simulink model "kundur_vsg"  (R2025b)
settings: Solver=ode23t  StartTime=0.0  StopTime=10.0  MaxStep=0.001  RelTol=1e-4
libraries: fl_lib x55, ee_lib x53, nesl_utility x17
(part 1 of 2)
settings Model: Creator=27443  LastModifiedBy=27443

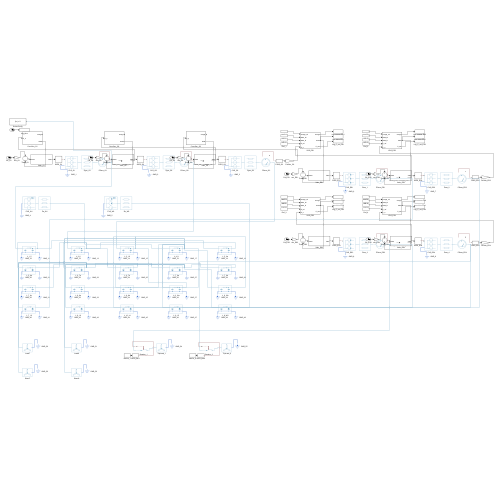
[thumbnail: Simulink's stored preview of the top-level diagram]
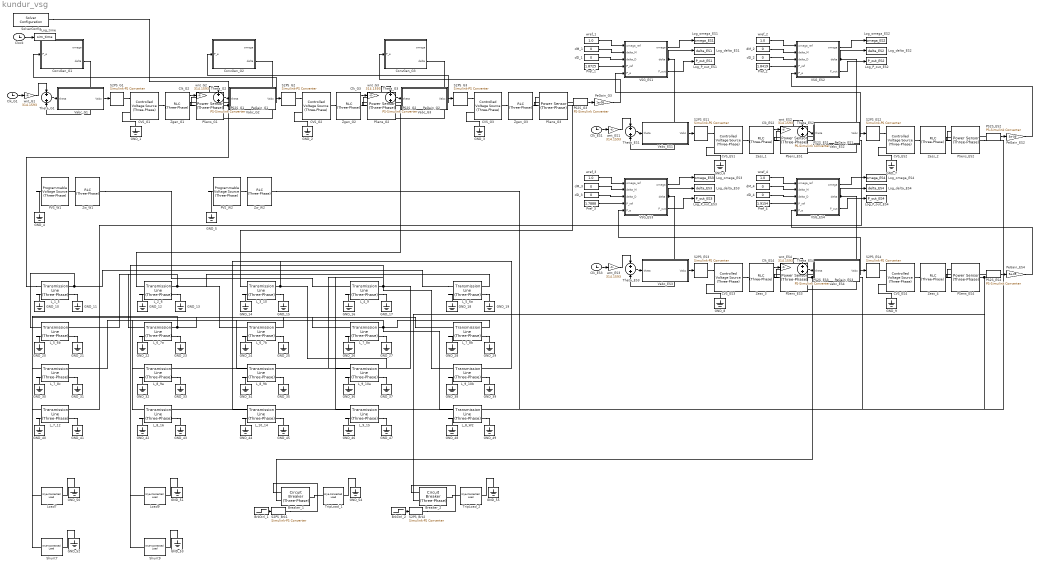
== system kundur_vsg ==
  Breaker_1 : ee_lib/Switches & Breakers/Circuit Breaker (Three-Phase)  R_closed=0.001 Ohm  G_open=1e-6 1/Ohm  threshold=0.5 V  breaker_behavior=ee.enum.switches.breakerBehavior.zeroCrossingEnable
      settings: InternalSimscapePortConfiguration="{\"Bottom\":[],\"Left\":[{\"id\":\"vT\",\"label\":\"vT\",\"type\":\"input\"},{\"id\":\"N1\",\"label\":\"~1\",\"type\":\"foundation.electrical.three_phase\"}],\"Right\":[{\"id\":\"N2\",\"label\":\"~2\",\"type\":\"foundation.electrical.three_phase\"}],\"Top\":[]}"
  Breaker_2 : ee_lib/Switches & Breakers/Circuit Breaker (Three-Phase)  R_closed=0.001 Ohm  G_open=1e-6 1/Ohm  threshold=0.5 V  breaker_behavior=ee.enum.switches.breakerBehavior.zeroCrossingEnable
      settings: InternalSimscapePortConfiguration="{\"Bottom\":[],\"Left\":[{\"id\":\"vT\",\"label\":\"vT\",\"type\":\"input\"},{\"id\":\"N1\",\"label\":\"~1\",\"type\":\"foundation.electrical.three_phase\"}],\"Right\":[{\"id\":\"N2\",\"label\":\"~2\",\"type\":\"foundation.electrical.three_phase\"}],\"Top\":[]}"
  BrkCtrl_1 : Step  Time=100  Before=1  After=0
  BrkCtrl_2 : Step  Time=100
  CVS_ES{1..4} (4 alike) : ee_lib/Sources/Controlled Voltage Source (Three-Phase)  input_option=ee.enum.inputType.instantaneous  FRated=60 Hz
      settings: InternalSimscapePortConfiguration="{\"Bottom\":[],\"Left\":[{\"id\":\"S\",\"label\":\"S\",\"type\":\"input\"},{\"id\":\"n\",\"label\":\"n\",\"type\":\"foundation.electrical.electrical\"}],\"Right\":[{\"id\":\"N\",\"label\":\"~\",\"type\":\"foundation.electrical.three_phase\"}],\"Top\":[]}"
  CVS_G1 : ee_lib/Sources/Controlled Voltage Source (Three-Phase)  input_option=ee.enum.inputType.instantaneous  FRated=60 Hz
      settings: InternalSimscapePortConfiguration="{\"Bottom\":[],\"Left\":[{\"id\":\"S\",\"label\":\"S\",\"type\":\"input\"},{\"id\":\"n\",\"label\":\"n\",\"type\":\"foundation.electrical.electrical\"}],\"Right\":[{\"id\":\"N\",\"label\":\"~\",\"type\":\"foundation.electrical.three_phase\"}],\"Top\":[]}"
  CVS_G2 : ee_lib/Sources/Controlled Voltage Source (Three-Phase)  input_option=ee.enum.inputType.instantaneous  FRated=60 Hz
      settings: InternalSimscapePortConfiguration="{\"Bottom\":[],\"Left\":[{\"id\":\"S\",\"label\":\"S\",\"type\":\"input\"},{\"id\":\"n\",\"label\":\"n\",\"type\":\"foundation.electrical.electrical\"}],\"Right\":[{\"id\":\"N\",\"label\":\"~\",\"type\":\"foundation.electrical.three_phase\"}],\"Top\":[]}"
  CVS_G3 : ee_lib/Sources/Controlled Voltage Source (Three-Phase)  input_option=ee.enum.inputType.instantaneous  FRated=60 Hz
      settings: InternalSimscapePortConfiguration="{\"Bottom\":[],\"Left\":[{\"id\":\"S\",\"label\":\"S\",\"type\":\"input\"},{\"id\":\"n\",\"label\":\"n\",\"type\":\"foundation.electrical.electrical\"}],\"Right\":[{\"id\":\"N\",\"label\":\"~\",\"type\":\"foundation.electrical.three_phase\"}],\"Top\":[]}"
  Clk_ES{1..4} (4 alike) : Clock
  Clk_G1 : Clock
  Clk_G2 : Clock
  Clk_G3 : Clock
  Clock : Clock
  ConvGen_G1 : Subsystem
  ConvGen_G2 : Subsystem
  ConvGen_G3 : Subsystem
  GND_{1..55} (55 alike) : fl_lib/Electrical/Electrical Elements/Electrical Reference
  L_10_14 : ee_lib/Passive/Lines/Transmission Line (Three-Phase)  length=1 km  freq=50 Hz  R=0.01 Ohm/km  L=0.5 mH/km  M=0.1 mH/km  Cl=9 uF/km  Cg=0.1 uF/km  Rm=0 Ohm/km  ModelTwoSections=ee.enum.enable.no  N=1  InterfacePosition=0.5 km  N1sec=1  N2sec=1  Access_ground=ee.enum.enable.no  R_parasitic=1e-6 Ohm  G_parasitic=1e-6 1/Ohm
      settings: InternalSimscapePortConfiguration="{\"Bottom\":[],\"Left\":[{\"id\":\"N1\",\"label\":\"~1\",\"type\":\"foundation.electrical.three_phase\"},{\"id\":\"g1\",\"label\":\"g1\",\"type\":\"foundation.electrical.electrical\"}],\"Right\":[{\"id\":\"N2\",\"label\":\"~2\",\"type\":\"foundation.electrical.three_phase\"},{\"id\":\"g2\",\"label\":\"g2\",\"type\":\"foundation.electrical.electrical\"}],\"Top\":[]}"
  L_1_5 : ee_lib/Passive/Lines/Transmission Line (Three-Phase)  length=5 km  freq=50 Hz  R=0.053 Ohm/km  L=1.41 mH/km  M=0.1 mH/km  Cl=9 uF/km  Cg=0.1 uF/km  Rm=0 Ohm/km  ModelTwoSections=ee.enum.enable.no  N=1  InterfacePosition=0.5 km  N1sec=1  N2sec=1  Access_ground=ee.enum.enable.no  R_parasitic=1e-6 Ohm  G_parasitic=1e-6 1/Ohm
      settings: InternalSimscapePortConfiguration="{\"Bottom\":[],\"Left\":[{\"id\":\"N1\",\"label\":\"~1\",\"type\":\"foundation.electrical.three_phase\"},{\"id\":\"g1\",\"label\":\"g1\",\"type\":\"foundation.electrical.electrical\"}],\"Right\":[{\"id\":\"N2\",\"label\":\"~2\",\"type\":\"foundation.electrical.three_phase\"},{\"id\":\"g2\",\"label\":\"g2\",\"type\":\"foundation.electrical.electrical\"}],\"Top\":[]}"
  L_2_6 : ee_lib/Passive/Lines/Transmission Line (Three-Phase)  length=5 km  freq=50 Hz  R=0.053 Ohm/km  L=1.41 mH/km  M=0.1 mH/km  Cl=9 uF/km  Cg=0.1 uF/km  Rm=0 Ohm/km  ModelTwoSections=ee.enum.enable.no  N=1  InterfacePosition=0.5 km  N1sec=1  N2sec=1  Access_ground=ee.enum.enable.no  R_parasitic=1e-6 Ohm  G_parasitic=1e-6 1/Ohm
      settings: InternalSimscapePortConfiguration="{\"Bottom\":[],\"Left\":[{\"id\":\"N1\",\"label\":\"~1\",\"type\":\"foundation.electrical.three_phase\"},{\"id\":\"g1\",\"label\":\"g1\",\"type\":\"foundation.electrical.electrical\"}],\"Right\":[{\"id\":\"N2\",\"label\":\"~2\",\"type\":\"foundation.electrical.three_phase\"},{\"id\":\"g2\",\"label\":\"g2\",\"type\":\"foundation.electrical.electrical\"}],\"Top\":[]}"
  L_3_10 : ee_lib/Passive/Lines/Transmission Line (Three-Phase)  length=5 km  freq=50 Hz  R=0.053 Ohm/km  L=1.41 mH/km  M=0.1 mH/km  Cl=9 uF/km  Cg=0.1 uF/km  Rm=0 Ohm/km  ModelTwoSections=ee.enum.enable.no  N=1  InterfacePosition=0.5 km  N1sec=1  N2sec=1  Access_ground=ee.enum.enable.no  R_parasitic=1e-6 Ohm  G_parasitic=1e-6 1/Ohm
      settings: InternalSimscapePortConfiguration="{\"Bottom\":[],\"Left\":[{\"id\":\"N1\",\"label\":\"~1\",\"type\":\"foundation.electrical.three_phase\"},{\"id\":\"g1\",\"label\":\"g1\",\"type\":\"foundation.electrical.electrical\"}],\"Right\":[{\"id\":\"N2\",\"label\":\"~2\",\"type\":\"foundation.electrical.three_phase\"},{\"id\":\"g2\",\"label\":\"g2\",\"type\":\"foundation.electrical.electrical\"}],\"Top\":[]}"
  L_4_9 : ee_lib/Passive/Lines/Transmission Line (Three-Phase)  length=5 km  freq=50 Hz  R=0.053 Ohm/km  L=1.41 mH/km  M=0.1 mH/km  Cl=9 uF/km  Cg=0.1 uF/km  Rm=0 Ohm/km  ModelTwoSections=ee.enum.enable.no  N=1  InterfacePosition=0.5 km  N1sec=1  N2sec=1  Access_ground=ee.enum.enable.no  R_parasitic=1e-6 Ohm  G_parasitic=1e-6 1/Ohm
      settings: InternalSimscapePortConfiguration="{\"Bottom\":[],\"Left\":[{\"id\":\"N1\",\"label\":\"~1\",\"type\":\"foundation.electrical.three_phase\"},{\"id\":\"g1\",\"label\":\"g1\",\"type\":\"foundation.electrical.electrical\"}],\"Right\":[{\"id\":\"N2\",\"label\":\"~2\",\"type\":\"foundation.electrical.three_phase\"},{\"id\":\"g2\",\"label\":\"g2\",\"type\":\"foundation.electrical.electrical\"}],\"Top\":[]}"
  L_5_6a : ee_lib/Passive/Lines/Transmission Line (Three-Phase)  length=25 km  freq=50 Hz  R=0.053 Ohm/km  L=1.41 mH/km  M=0.1 mH/km  Cl=9 uF/km  Cg=0.1 uF/km  Rm=0 Ohm/km  ModelTwoSections=ee.enum.enable.no  N=1  InterfacePosition=0.5 km  N1sec=1  N2sec=1  Access_ground=ee.enum.enable.no  R_parasitic=1e-6 Ohm  G_parasitic=1e-6 1/Ohm
      settings: InternalSimscapePortConfiguration="{\"Bottom\":[],\"Left\":[{\"id\":\"N1\",\"label\":\"~1\",\"type\":\"foundation.electrical.three_phase\"},{\"id\":\"g1\",\"label\":\"g1\",\"type\":\"foundation.electrical.electrical\"}],\"Right\":[{\"id\":\"N2\",\"label\":\"~2\",\"type\":\"foundation.electrical.three_phase\"},{\"id\":\"g2\",\"label\":\"g2\",\"type\":\"foundation.electrical.electrical\"}],\"Top\":[]}"
  L_5_6b : ee_lib/Passive/Lines/Transmission Line (Three-Phase)  length=25 km  freq=50 Hz  R=0.053 Ohm/km  L=1.41 mH/km  M=0.1 mH/km  Cl=9 uF/km  Cg=0.1 uF/km  Rm=0 Ohm/km  ModelTwoSections=ee.enum.enable.no  N=1  InterfacePosition=0.5 km  N1sec=1  N2sec=1  Access_ground=ee.enum.enable.no  R_parasitic=1e-6 Ohm  G_parasitic=1e-6 1/Ohm
      settings: InternalSimscapePortConfiguration="{\"Bottom\":[],\"Left\":[{\"id\":\"N1\",\"label\":\"~1\",\"type\":\"foundation.electrical.three_phase\"},{\"id\":\"g1\",\"label\":\"g1\",\"type\":\"foundation.electrical.electrical\"}],\"Right\":[{\"id\":\"N2\",\"label\":\"~2\",\"type\":\"foundation.electrical.three_phase\"},{\"id\":\"g2\",\"label\":\"g2\",\"type\":\"foundation.electrical.electrical\"}],\"Top\":[]}"
  L_6_7a : ee_lib/Passive/Lines/Transmission Line (Three-Phase)  length=10 km  freq=50 Hz  R=0.053 Ohm/km  L=1.41 mH/km  M=0.1 mH/km  Cl=9 uF/km  Cg=0.1 uF/km  Rm=0 Ohm/km  ModelTwoSections=ee.enum.enable.no  N=1  InterfacePosition=0.5 km  N1sec=1  N2sec=1  Access_ground=ee.enum.enable.no  R_parasitic=1e-6 Ohm  G_parasitic=1e-6 1/Ohm
      settings: InternalSimscapePortConfiguration="{\"Bottom\":[],\"Left\":[{\"id\":\"N1\",\"label\":\"~1\",\"type\":\"foundation.electrical.three_phase\"},{\"id\":\"g1\",\"label\":\"g1\",\"type\":\"foundation.electrical.electrical\"}],\"Right\":[{\"id\":\"N2\",\"label\":\"~2\",\"type\":\"foundation.electrical.three_phase\"},{\"id\":\"g2\",\"label\":\"g2\",\"type\":\"foundation.electrical.electrical\"}],\"Top\":[]}"
  L_6_7b : ee_lib/Passive/Lines/Transmission Line (Three-Phase)  length=10 km  freq=50 Hz  R=0.053 Ohm/km  L=1.41 mH/km  M=0.1 mH/km  Cl=9 uF/km  Cg=0.1 uF/km  Rm=0 Ohm/km  ModelTwoSections=ee.enum.enable.no  N=1  InterfacePosition=0.5 km  N1sec=1  N2sec=1  Access_ground=ee.enum.enable.no  R_parasitic=1e-6 Ohm  G_parasitic=1e-6 1/Ohm
      settings: InternalSimscapePortConfiguration="{\"Bottom\":[],\"Left\":[{\"id\":\"N1\",\"label\":\"~1\",\"type\":\"foundation.electrical.three_phase\"},{\"id\":\"g1\",\"label\":\"g1\",\"type\":\"foundation.electrical.electrical\"}],\"Right\":[{\"id\":\"N2\",\"label\":\"~2\",\"type\":\"foundation.electrical.three_phase\"},{\"id\":\"g2\",\"label\":\"g2\",\"type\":\"foundation.electrical.electrical\"}],\"Top\":[]}"
  L_7_12 : ee_lib/Passive/Lines/Transmission Line (Three-Phase)  length=1 km  freq=50 Hz  R=0.01 Ohm/km  L=0.5 mH/km  M=0.1 mH/km  Cl=9 uF/km  Cg=0.1 uF/km  Rm=0 Ohm/km  ModelTwoSections=ee.enum.enable.no  N=1  InterfacePosition=0.5 km  N1sec=1  N2sec=1  Access_ground=ee.enum.enable.no  R_parasitic=1e-6 Ohm  G_parasitic=1e-6 1/Ohm
      settings: InternalSimscapePortConfiguration="{\"Bottom\":[],\"Left\":[{\"id\":\"N1\",\"label\":\"~1\",\"type\":\"foundation.electrical.three_phase\"},{\"id\":\"g1\",\"label\":\"g1\",\"type\":\"foundation.electrical.electrical\"}],\"Right\":[{\"id\":\"N2\",\"label\":\"~2\",\"type\":\"foundation.electrical.three_phase\"},{\"id\":\"g2\",\"label\":\"g2\",\"type\":\"foundation.electrical.electrical\"}],\"Top\":[]}"
  L_7_8a : ee_lib/Passive/Lines/Transmission Line (Three-Phase)  length=110 km  freq=50 Hz  R=0.053 Ohm/km  L=1.41 mH/km  M=0.1 mH/km  Cl=9 uF/km  Cg=0.1 uF/km  Rm=0 Ohm/km  ModelTwoSections=ee.enum.enable.no  N=1  InterfacePosition=0.5 km  N1sec=1  N2sec=1  Access_ground=ee.enum.enable.no  R_parasitic=1e-6 Ohm  G_parasitic=1e-6 1/Ohm
      settings: InternalSimscapePortConfiguration="{\"Bottom\":[],\"Left\":[{\"id\":\"N1\",\"label\":\"~1\",\"type\":\"foundation.electrical.three_phase\"},{\"id\":\"g1\",\"label\":\"g1\",\"type\":\"foundation.electrical.electrical\"}],\"Right\":[{\"id\":\"N2\",\"label\":\"~2\",\"type\":\"foundation.electrical.three_phase\"},{\"id\":\"g2\",\"label\":\"g2\",\"type\":\"foundation.electrical.electrical\"}],\"Top\":[]}"
  L_7_8b : ee_lib/Passive/Lines/Transmission Line (Three-Phase)  length=110 km  freq=50 Hz  R=0.053 Ohm/km  L=1.41 mH/km  M=0.1 mH/km  Cl=9 uF/km  Cg=0.1 uF/km  Rm=0 Ohm/km  ModelTwoSections=ee.enum.enable.no  N=1  InterfacePosition=0.5 km  N1sec=1  N2sec=1  Access_ground=ee.enum.enable.no  R_parasitic=1e-6 Ohm  G_parasitic=1e-6 1/Ohm
      settings: InternalSimscapePortConfiguration="{\"Bottom\":[],\"Left\":[{\"id\":\"N1\",\"label\":\"~1\",\"type\":\"foundation.electrical.three_phase\"},{\"id\":\"g1\",\"label\":\"g1\",\"type\":\"foundation.electrical.electrical\"}],\"Right\":[{\"id\":\"N2\",\"label\":\"~2\",\"type\":\"foundation.electrical.three_phase\"},{\"id\":\"g2\",\"label\":\"g2\",\"type\":\"foundation.electrical.electrical\"}],\"Top\":[]}"
  L_7_8c : ee_lib/Passive/Lines/Transmission Line (Three-Phase)  length=110 km  freq=50 Hz  R=0.053 Ohm/km  L=1.41 mH/km  M=0.1 mH/km  Cl=9 uF/km  Cg=0.1 uF/km  Rm=0 Ohm/km  ModelTwoSections=ee.enum.enable.no  N=1  InterfacePosition=0.5 km  N1sec=1  N2sec=1  Access_ground=ee.enum.enable.no  R_parasitic=1e-6 Ohm  G_parasitic=1e-6 1/Ohm
      settings: InternalSimscapePortConfiguration="{\"Bottom\":[],\"Left\":[{\"id\":\"N1\",\"label\":\"~1\",\"type\":\"foundation.electrical.three_phase\"},{\"id\":\"g1\",\"label\":\"g1\",\"type\":\"foundation.electrical.electrical\"}],\"Right\":[{\"id\":\"N2\",\"label\":\"~2\",\"type\":\"foundation.electrical.three_phase\"},{\"id\":\"g2\",\"label\":\"g2\",\"type\":\"foundation.electrical.electrical\"}],\"Top\":[]}"
  L_8_16 : ee_lib/Passive/Lines/Transmission Line (Three-Phase)  length=1 km  freq=50 Hz  R=0.01 Ohm/km  L=0.5 mH/km  M=0.1 mH/km  Cl=9 uF/km  Cg=0.1 uF/km  Rm=0 Ohm/km  ModelTwoSections=ee.enum.enable.no  N=1  InterfacePosition=0.5 km  N1sec=1  N2sec=1  Access_ground=ee.enum.enable.no  R_parasitic=1e-6 Ohm  G_parasitic=1e-6 1/Ohm
      settings: InternalSimscapePortConfiguration="{\"Bottom\":[],\"Left\":[{\"id\":\"N1\",\"label\":\"~1\",\"type\":\"foundation.electrical.three_phase\"},{\"id\":\"g1\",\"label\":\"g1\",\"type\":\"foundation.electrical.electrical\"}],\"Right\":[{\"id\":\"N2\",\"label\":\"~2\",\"type\":\"foundation.electrical.three_phase\"},{\"id\":\"g2\",\"label\":\"g2\",\"type\":\"foundation.electrical.electrical\"}],\"Top\":[]}"
  L_8_9a : ee_lib/Passive/Lines/Transmission Line (Three-Phase)  length=10 km  freq=50 Hz  R=0.053 Ohm/km  L=1.41 mH/km  M=0.1 mH/km  Cl=9 uF/km  Cg=0.1 uF/km  Rm=0 Ohm/km  ModelTwoSections=ee.enum.enable.no  N=1  InterfacePosition=0.5 km  N1sec=1  N2sec=1  Access_ground=ee.enum.enable.no  R_parasitic=1e-6 Ohm  G_parasitic=1e-6 1/Ohm
      settings: InternalSimscapePortConfiguration="{\"Bottom\":[],\"Left\":[{\"id\":\"N1\",\"label\":\"~1\",\"type\":\"foundation.electrical.three_phase\"},{\"id\":\"g1\",\"label\":\"g1\",\"type\":\"foundation.electrical.electrical\"}],\"Right\":[{\"id\":\"N2\",\"label\":\"~2\",\"type\":\"foundation.electrical.three_phase\"},{\"id\":\"g2\",\"label\":\"g2\",\"type\":\"foundation.electrical.electrical\"}],\"Top\":[]}"
  L_8_9b : ee_lib/Passive/Lines/Transmission Line (Three-Phase)  length=10 km  freq=50 Hz  R=0.053 Ohm/km  L=1.41 mH/km  M=0.1 mH/km  Cl=9 uF/km  Cg=0.1 uF/km  Rm=0 Ohm/km  ModelTwoSections=ee.enum.enable.no  N=1  InterfacePosition=0.5 km  N1sec=1  N2sec=1  Access_ground=ee.enum.enable.no  R_parasitic=1e-6 Ohm  G_parasitic=1e-6 1/Ohm
      settings: InternalSimscapePortConfiguration="{\"Bottom\":[],\"Left\":[{\"id\":\"N1\",\"label\":\"~1\",\"type\":\"foundation.electrical.three_phase\"},{\"id\":\"g1\",\"label\":\"g1\",\"type\":\"foundation.electrical.electrical\"}],\"Right\":[{\"id\":\"N2\",\"label\":\"~2\",\"type\":\"foundation.electrical.three_phase\"},{\"id\":\"g2\",\"label\":\"g2\",\"type\":\"foundation.electrical.electrical\"}],\"Top\":[]}"
  L_8_W2 : ee_lib/Passive/Lines/Transmission Line (Three-Phase)  length=1 km  freq=50 Hz  R=0.01 Ohm/km  L=0.5 mH/km  M=0.1 mH/km  Cl=9 uF/km  Cg=0.1 uF/km  Rm=0 Ohm/km  ModelTwoSections=ee.enum.enable.no  N=1  InterfacePosition=0.5 km  N1sec=1  N2sec=1  Access_ground=ee.enum.enable.no  R_parasitic=1e-6 Ohm  G_parasitic=1e-6 1/Ohm
      settings: InternalSimscapePortConfiguration="{\"Bottom\":[],\"Left\":[{\"id\":\"N1\",\"label\":\"~1\",\"type\":\"foundation.electrical.three_phase\"},{\"id\":\"g1\",\"label\":\"g1\",\"type\":\"foundation.electrical.electrical\"}],\"Right\":[{\"id\":\"N2\",\"label\":\"~2\",\"type\":\"foundation.electrical.three_phase\"},{\"id\":\"g2\",\"label\":\"g2\",\"type\":\"foundation.electrical.electrical\"}],\"Top\":[]}"
  L_9_10a : ee_lib/Passive/Lines/Transmission Line (Three-Phase)  length=25 km  freq=50 Hz  R=0.053 Ohm/km  L=1.41 mH/km  M=0.1 mH/km  Cl=9 uF/km  Cg=0.1 uF/km  Rm=0 Ohm/km  ModelTwoSections=ee.enum.enable.no  N=1  InterfacePosition=0.5 km  N1sec=1  N2sec=1  Access_ground=ee.enum.enable.no  R_parasitic=1e-6 Ohm  G_parasitic=1e-6 1/Ohm
      settings: InternalSimscapePortConfiguration="{\"Bottom\":[],\"Left\":[{\"id\":\"N1\",\"label\":\"~1\",\"type\":\"foundation.electrical.three_phase\"},{\"id\":\"g1\",\"label\":\"g1\",\"type\":\"foundation.electrical.electrical\"}],\"Right\":[{\"id\":\"N2\",\"label\":\"~2\",\"type\":\"foundation.electrical.three_phase\"},{\"id\":\"g2\",\"label\":\"g2\",\"type\":\"foundation.electrical.electrical\"}],\"Top\":[]}"
  L_9_10b : ee_lib/Passive/Lines/Transmission Line (Three-Phase)  length=25 km  freq=50 Hz  R=0.053 Ohm/km  L=1.41 mH/km  M=0.1 mH/km  Cl=9 uF/km  Cg=0.1 uF/km  Rm=0 Ohm/km  ModelTwoSections=ee.enum.enable.no  N=1  InterfacePosition=0.5 km  N1sec=1  N2sec=1  Access_ground=ee.enum.enable.no  R_parasitic=1e-6 Ohm  G_parasitic=1e-6 1/Ohm
      settings: InternalSimscapePortConfiguration="{\"Bottom\":[],\"Left\":[{\"id\":\"N1\",\"label\":\"~1\",\"type\":\"foundation.electrical.three_phase\"},{\"id\":\"g1\",\"label\":\"g1\",\"type\":\"foundation.electrical.electrical\"}],\"Right\":[{\"id\":\"N2\",\"label\":\"~2\",\"type\":\"foundation.electrical.three_phase\"},{\"id\":\"g2\",\"label\":\"g2\",\"type\":\"foundation.electrical.electrical\"}],\"Top\":[]}"
  L_9_15 : ee_lib/Passive/Lines/Transmission Line (Three-Phase)  length=1 km  freq=50 Hz  R=0.01 Ohm/km  L=0.5 mH/km  M=0.1 mH/km  Cl=9 uF/km  Cg=0.1 uF/km  Rm=0 Ohm/km  ModelTwoSections=ee.enum.enable.no  N=1  InterfacePosition=0.5 km  N1sec=1  N2sec=1  Access_ground=ee.enum.enable.no  R_parasitic=1e-6 Ohm  G_parasitic=1e-6 1/Ohm
      settings: InternalSimscapePortConfiguration="{\"Bottom\":[],\"Left\":[{\"id\":\"N1\",\"label\":\"~1\",\"type\":\"foundation.electrical.three_phase\"},{\"id\":\"g1\",\"label\":\"g1\",\"type\":\"foundation.electrical.electrical\"}],\"Right\":[{\"id\":\"N2\",\"label\":\"~2\",\"type\":\"foundation.electrical.three_phase\"},{\"id\":\"g2\",\"label\":\"g2\",\"type\":\"foundation.electrical.electrical\"}],\"Top\":[]}"
  Load7 : ee_lib/Passive/RLC Assemblies/Wye-Connected Load  port_option=ee.enum.threePhasePort.composite  parameterization=2  component_structure=4  component_structure_PQ=ee.enum.rlc.structure.R  R=1 Ohm  L=1e-3 H  C=1e-6 F  VRated=230000 V  FRated=50 Hz  P=967000000 W  Qpos=100000000 A*V  Qneg=-1e2 A*V  R_parasitic=0 Ohm  G_parasitic=0 1/Ohm  R_parasitic_PQ=0 Ohm  G_parasitic_PQ=0 1/Ohm  Vmag0=24e3 V  Vang0=0 deg  Freq0=60 Hz  IL_specify=off  IL_priority=High  IL=[0, 0, 0] A  IL_nominal_specify=off  IL_nominal_value=1  IL_nominal_unit=A  VC_specify=off  VC_priority=High  VC=[0, 0, 0] V  VC_nominal_specify=off  VC_nominal_value=1  VC_nominal_unit=V
  Load9 : ee_lib/Passive/RLC Assemblies/Wye-Connected Load  port_option=ee.enum.threePhasePort.composite  parameterization=2  component_structure=4  component_structure_PQ=ee.enum.rlc.structure.R  R=1 Ohm  L=1e-3 H  C=1e-6 F  VRated=230000 V  FRated=50 Hz  P=1767000000 W  Qpos=100000000 A*V  Qneg=-1e2 A*V  R_parasitic=0 Ohm  G_parasitic=0 1/Ohm  R_parasitic_PQ=0 Ohm  G_parasitic_PQ=0 1/Ohm  Vmag0=24e3 V  Vang0=0 deg  Freq0=60 Hz  IL_specify=off  IL_priority=High  IL=[0, 0, 0] A  IL_nominal_specify=off  IL_nominal_value=1  IL_nominal_unit=A  VC_specify=off  VC_priority=High  VC=[0, 0, 0] V  VC_nominal_specify=off  VC_nominal_value=1  VC_nominal_unit=V
  Log_P_out_ES1 : ToWorkspace  VariableName=P_out_ES1  SaveFormat=Timeseries
  Log_P_out_ES2 : ToWorkspace  VariableName=P_out_ES2  SaveFormat=Timeseries
  Log_P_out_ES3 : ToWorkspace  VariableName=P_out_ES3  SaveFormat=Timeseries
  Log_P_out_ES4 : ToWorkspace  VariableName=P_out_ES4  SaveFormat=Timeseries
  Log_delta_ES1 : ToWorkspace  VariableName=delta_ES1  SaveFormat=Timeseries
  Log_delta_ES2 : ToWorkspace  VariableName=delta_ES2  SaveFormat=Timeseries
  Log_delta_ES3 : ToWorkspace  VariableName=delta_ES3  SaveFormat=Timeseries
  Log_delta_ES4 : ToWorkspace  VariableName=delta_ES4  SaveFormat=Timeseries
  Log_omega_ES1 : ToWorkspace  VariableName=omega_ES1  SaveFormat=Timeseries
  Log_omega_ES2 : ToWorkspace  VariableName=omega_ES2  SaveFormat=Timeseries
  Log_omega_ES3 : ToWorkspace  VariableName=omega_ES3  SaveFormat=Timeseries
  Log_omega_ES4 : ToWorkspace  VariableName=omega_ES4  SaveFormat=Timeseries
  Log_time : ToWorkspace  VariableName=sim_time  SaveFormat=Timeseries
  PS2S_ES{1..4} (4 alike) : nesl_utility/PS-Simulink Converter  PhysicalDomain=network_engine_domain  SubClassName=ps_output  LeftPortType=input  RightPortType=output  PseudoPeriodic=off  Frequencies=[]  VectorFormat=inherit  Unit=inherit  AffineConversion=off
  PS2S_G1 : nesl_utility/PS-Simulink Converter  PhysicalDomain=network_engine_domain  SubClassName=ps_output  LeftPortType=input  RightPortType=output  PseudoPeriodic=off  Frequencies=[]  VectorFormat=inherit  Unit=inherit  AffineConversion=off
  PS2S_G2 : nesl_utility/PS-Simulink Converter  PhysicalDomain=network_engine_domain  SubClassName=ps_output  LeftPortType=input  RightPortType=output  PseudoPeriodic=off  Frequencies=[]  VectorFormat=inherit  Unit=inherit  AffineConversion=off
  PS2S_G3 : nesl_utility/PS-Simulink Converter  PhysicalDomain=network_engine_domain  SubClassName=ps_output  LeftPortType=input  RightPortType=output  PseudoPeriodic=off  Frequencies=[]  VectorFormat=inherit  Unit=inherit  AffineConversion=off
  PSens_ES{1..4} (4 alike) : ee_lib/Sensors & Transducers/Power Sensor (Three-Phase)  load_type=ee.enum.passive.type_balanced.balanced  f0=60 Hz
      settings: InternalSimscapePortConfiguration="{\"Bottom\":[],\"Left\":[{\"id\":\"N1\",\"label\":\"~1\",\"type\":\"foundation.electrical.three_phase\"}],\"Right\":[{\"id\":\"N2\",\"label\":\"~2\",\"type\":\"foundation.electrical.three_phase\"}],\"Top\":[{\"id\":\"Pm\",\"label\":\"P\",\"type\":\"output\"},{\"id\":\"Qm\",\"label\":\"Q\",\"type\":\"output\"}]}"
  PSens_G1 : ee_lib/Sensors & Transducers/Power Sensor (Three-Phase)  load_type=ee.enum.passive.type_balanced.balanced  f0=60 Hz
      settings: InternalSimscapePortConfiguration="{\"Bottom\":[],\"Left\":[{\"id\":\"N1\",\"label\":\"~1\",\"type\":\"foundation.electrical.three_phase\"}],\"Right\":[{\"id\":\"N2\",\"label\":\"~2\",\"type\":\"foundation.electrical.three_phase\"}],\"Top\":[{\"id\":\"Pm\",\"label\":\"P\",\"type\":\"output\"},{\"id\":\"Qm\",\"label\":\"Q\",\"type\":\"output\"}]}"
  PSens_G2 : ee_lib/Sensors & Transducers/Power Sensor (Three-Phase)  load_type=ee.enum.passive.type_balanced.balanced  f0=60 Hz
      settings: InternalSimscapePortConfiguration="{\"Bottom\":[],\"Left\":[{\"id\":\"N1\",\"label\":\"~1\",\"type\":\"foundation.electrical.three_phase\"}],\"Right\":[{\"id\":\"N2\",\"label\":\"~2\",\"type\":\"foundation.electrical.three_phase\"}],\"Top\":[{\"id\":\"Pm\",\"label\":\"P\",\"type\":\"output\"},{\"id\":\"Qm\",\"label\":\"Q\",\"type\":\"output\"}]}"
  PSens_G3 : ee_lib/Sensors & Transducers/Power Sensor (Three-Phase)  load_type=ee.enum.passive.type_balanced.balanced  f0=60 Hz
      settings: InternalSimscapePortConfiguration="{\"Bottom\":[],\"Left\":[{\"id\":\"N1\",\"label\":\"~1\",\"type\":\"foundation.electrical.three_phase\"}],\"Right\":[{\"id\":\"N2\",\"label\":\"~2\",\"type\":\"foundation.electrical.three_phase\"}],\"Top\":[{\"id\":\"Pm\",\"label\":\"P\",\"type\":\"output\"},{\"id\":\"Qm\",\"label\":\"Q\",\"type\":\"output\"}]}"
  PVS_W1 : ee_lib/Sources/Programmable Voltage Source (Three-Phase)  magnitude_type=ee.enum.timechanging.constant  vline_rms=230000 V  magn_ramp=1 V/s  magn_step=1 V  magn_modu_magn=1 V  magn_modu_freq=1 Hz  magn_t1=1 s  magn_t2=2 s  frequency_type=ee.enum.timechanging.constant  freq=50 Hz  freq_ramp=1 Hz/s  freq_step=1 Hz  freq_modu_magn=1 Hz  freq_modu_freq=1 Hz  freq_t1=1 s  freq_t2=2 s  phase_type=ee.enum.timechanging.constant  shift=-1 deg  phase_ramp=1 deg/s  phase_step=1 deg  phase_modu_magn=1 deg  phase_modu_freq=1 Hz  phase_t1=1 s  phase_t2=2 s  impedance_option=1  SShortCircuit=1e6 A*V  XR=15  R=0.01 Ohm  L=3.97e-4 H  G_parasitic=1e-6 1/Ohm  harmonic_option=0  harmonic_orders=[5, 7, 11, 13]  harmonic_ratios=[.1, .1, .1, .1]  harmonic_shifts=[0, 0, 0, 0] deg  harmonic_sequences=[1, 1, 1, 1]  harmonic_t1=-inf s  harmonic_t2=inf s  I_specify=off  I_priority=None  I=[0, 0, 0] A  I_nominal_specify=off  I_nominal_value=1  I_nominal_unit=A  V_specify=off  V_priority=None  V=[0, 0, 0] V  V_nominal_specify=off  V_nominal_value=1  V_nominal_unit=V
      settings: InternalSimscapePortConfiguration="{\"Bottom\":[],\"Left\":[{\"id\":\"n\",\"label\":\"n\",\"type\":\"foundation.electrical.electrical\"}],\"Right\":[{\"id\":\"N\",\"label\":\"~\",\"type\":\"foundation.electrical.three_phase\"}],\"Top\":[]}"
  PVS_W2 : ee_lib/Sources/Programmable Voltage Source (Three-Phase)  magnitude_type=ee.enum.timechanging.constant  vline_rms=230000 V  magn_ramp=1 V/s  magn_step=1 V  magn_modu_magn=1 V  magn_modu_freq=1 Hz  magn_t1=1 s  magn_t2=2 s  frequency_type=ee.enum.timechanging.constant  freq=50 Hz  freq_ramp=1 Hz/s  freq_step=1 Hz  freq_modu_magn=1 Hz  freq_modu_freq=1 Hz  freq_t1=1 s  freq_t2=2 s  phase_type=ee.enum.timechanging.constant  shift=-4 deg  phase_ramp=1 deg/s  phase_step=1 deg  phase_modu_magn=1 deg  phase_modu_freq=1 Hz  phase_t1=1 s  phase_t2=2 s  impedance_option=1  SShortCircuit=1e6 A*V  XR=15  R=0.01 Ohm  L=3.97e-4 H  G_parasitic=1e-6 1/Ohm  harmonic_option=0  harmonic_orders=[5, 7, 11, 13]  harmonic_ratios=[.1, .1, .1, .1]  harmonic_shifts=[0, 0, 0, 0] deg  harmonic_sequences=[1, 1, 1, 1]  harmonic_t1=-inf s  harmonic_t2=inf s  I_specify=off  I_priority=None  I=[0, 0, 0] A  I_nominal_specify=off  I_nominal_value=1  I_nominal_unit=A  V_specify=off  V_priority=None  V=[0, 0, 0] V  V_nominal_specify=off  V_nominal_value=1  V_nominal_unit=V
      settings: InternalSimscapePortConfiguration="{\"Bottom\":[],\"Left\":[{\"id\":\"n\",\"label\":\"n\",\"type\":\"foundation.electrical.electrical\"}],\"Right\":[{\"id\":\"N\",\"label\":\"~\",\"type\":\"foundation.electrical.three_phase\"}],\"Top\":[]}"
  PeGain_ES{1..4} (4 alike) : Gain  Gain=5e-09
  PeGain_G1 : Gain  Gain=1e-08
  PeGain_G2 : Gain  Gain=1e-08
  PeGain_G3 : Gain  Gain=1e-08
  Pref_1 : Constant  Value=1.8725
  Pref_2 : Constant  Value=1.8419
  Pref_3 : Constant  Value=1.7888
  Pref_4 : Constant  Value=1.9154
  S2PS_Brk1 : nesl_utility/Simulink-PS Converter  PhysicalDomain=network_engine_domain  SubClassName=ps_input  LeftPortType=input  RightPortType=output  PseudoPeriodic=off  Frequencies=[]  NoiseDistribution=none  NoiseParameters=[]  Unit=1  AffineConversion=off  FilteringAndDerivatives=provide  SimscapeFilterOrder=1  InputFilterTimeConstant=0.001  UdotUserProvided=0
  S2PS_Brk2 : nesl_utility/Simulink-PS Converter  PhysicalDomain=network_engine_domain  SubClassName=ps_input  LeftPortType=input  RightPortType=output  PseudoPeriodic=off  Frequencies=[]  NoiseDistribution=none  NoiseParameters=[]  Unit=1  AffineConversion=off  FilteringAndDerivatives=provide  SimscapeFilterOrder=1  InputFilterTimeConstant=0.001  UdotUserProvided=0
  S2PS_ES{1..4} (4 alike) : nesl_utility/Simulink-PS Converter  PhysicalDomain=network_engine_domain  SubClassName=ps_input  LeftPortType=input  RightPortType=output  PseudoPeriodic=off  Frequencies=[]  NoiseDistribution=none  NoiseParameters=[]  Unit=1  AffineConversion=off  FilteringAndDerivatives=provide  SimscapeFilterOrder=1  InputFilterTimeConstant=0.001  UdotUserProvided=0
  S2PS_G1 : nesl_utility/Simulink-PS Converter  PhysicalDomain=network_engine_domain  SubClassName=ps_input  LeftPortType=input  RightPortType=output  PseudoPeriodic=off  Frequencies=[]  NoiseDistribution=none  NoiseParameters=[]  Unit=1  AffineConversion=off  FilteringAndDerivatives=provide  SimscapeFilterOrder=1  InputFilterTimeConstant=0.001  UdotUserProvided=0
  S2PS_G2 : nesl_utility/Simulink-PS Converter  PhysicalDomain=network_engine_domain  SubClassName=ps_input  LeftPortType=input  RightPortType=output  PseudoPeriodic=off  Frequencies=[]  NoiseDistribution=none  NoiseParameters=[]  Unit=1  AffineConversion=off  FilteringAndDerivatives=provide  SimscapeFilterOrder=1  InputFilterTimeConstant=0.001  UdotUserProvided=0
  S2PS_G3 : nesl_utility/Simulink-PS Converter  PhysicalDomain=network_engine_domain  SubClassName=ps_input  LeftPortType=input  RightPortType=output  PseudoPeriodic=off  Frequencies=[]  NoiseDistribution=none  NoiseParameters=[]  Unit=1  AffineConversion=off  FilteringAndDerivatives=provide  SimscapeFilterOrder=1  InputFilterTimeConstant=0.001  UdotUserProvided=0
  Shunt7 : ee_lib/Passive/RLC Assemblies/Wye-Connected Load  port_option=ee.enum.threePhasePort.composite  parameterization=2  component_structure=3  component_structure_PQ=ee.enum.rlc.structure.R  R=1 Ohm  L=1e-3 H  C=1e-6 F  VRated=230000 V  FRated=50 Hz  P=1e3 W  Qpos=1e2 A*V  Qneg=200000000 A*V  R_parasitic=0 Ohm  G_parasitic=0 1/Ohm  R_parasitic_PQ=0 Ohm  G_parasitic_PQ=0 1/Ohm  Vmag0=24e3 V  Vang0=0 deg  Freq0=60 Hz  IL_specify=off  IL_priority=High  IL=[0, 0, 0] A  IL_nominal_specify=off  IL_nominal_value=1  IL_nominal_unit=A  VC_specify=off  VC_priority=High  VC=[0, 0, 0] V  VC_nominal_specify=off  VC_nominal_value=1  VC_nominal_unit=V
  Shunt9 : ee_lib/Passive/RLC Assemblies/Wye-Connected Load  port_option=ee.enum.threePhasePort.composite  parameterization=2  component_structure=3  component_structure_PQ=ee.enum.rlc.structure.R  R=1 Ohm  L=1e-3 H  C=1e-6 F  VRated=230000 V  FRated=50 Hz  P=1e3 W  Qpos=1e2 A*V  Qneg=350000000 A*V  R_parasitic=0 Ohm  G_parasitic=0 1/Ohm  R_parasitic_PQ=0 Ohm  G_parasitic_PQ=0 1/Ohm  Vmag0=24e3 V  Vang0=0 deg  Freq0=60 Hz  IL_specify=off  IL_priority=High  IL=[0, 0, 0] A  IL_nominal_specify=off  IL_nominal_value=1  IL_nominal_unit=A  VC_specify=off  VC_priority=High  VC=[0, 0, 0] V  VC_nominal_specify=off  VC_nominal_value=1  VC_nominal_unit=V
  SolverConfig : nesl_utility/Solver Configuration  PhysicalDomain=network_engine_domain  SubClassName=solver  LeftPortType=input  RightPortType=generic  Tones=[]  Harmonics=[]  SimulateNoise=off  Profile=off  UseLocalSampling=off  EnableSwitchedLinearOptims=on  FrequencyDomain=off  UseCCode=off  RelTol=0.001  AbsTol=0.001  MinStep=1e-09  ToWorkspace=off  RevertToSquareIcSolve=off  NumHomotopyIterations=100  PhasorMode=off  PhasorModeNumHarmonics=1  ConsistencySolver=NEWTON_XTOL_AFTER_FTOL  IndexReductionMethod=DerivativeReplacement  DoDC=off  ResidualTolerance=1e-09  ConsistencyTolSource=GLOBAL  ConsistencyAbsTol=0.001  ConsistencyRelTol=0.001  ConsistencyTolFactor=0.001  UseLocalSolver=off  LocalSolverChoice=NE_BACKWARD_EULER_ADVANCER  ResolveIndetEquations=on  FunctionEvalNumThread=1  LocalSolverSampleTime=0.001  DoFixedCost=off  MaxNonlinIter=3  MaxModeIter=2  ComputeImpulses=off  ImpulseIterations=2  LinearAlgebra=auto  LinearAlgebraNumThread=0  EquationFormulation=NE_TIME_EF  DelaysMemoryBudget=1024  AutomaticFiltering=on  FilteringTimeConstant=0.001  PartitionStorageMethod=AS_NEEDED  PartitionMemoryBudget=1024  PartitionMethod=ROBUST  MultibodyUseLocalSolver=off  MultibodyLocalSolverChoice=ODE1  MultibodyLocalSolverSampleTime=0.001
  Theta_ES{1..4} (4 alike) : Sum
  Theta_G1 : Sum
  Theta_G2 : Sum
  Theta_G3 : Sum
  TripLoad_1 : ee_lib/Passive/RLC Assemblies/Wye-Connected Load  port_option=ee.enum.threePhasePort.composite  parameterization=2  component_structure=1  component_structure_PQ=ee.enum.rlc.structure.R  R=1 Ohm  L=1e-3 H  C=1e-6 F  VRated=230000 V  FRated=50 Hz  P=248000000 W  Qpos=1e2 A*V  Qneg=-1e2 A*V  R_parasitic=0 Ohm  G_parasitic=0 1/Ohm  R_parasitic_PQ=0 Ohm  G_parasitic_PQ=0 1/Ohm  Vmag0=24e3 V  Vang0=0 deg  Freq0=60 Hz  IL_specify=off  IL_priority=High  IL=[0, 0, 0] A  IL_nominal_specify=off  IL_nominal_value=1  IL_nominal_unit=A  VC_specify=off  VC_priority=High  VC=[0, 0, 0] V  VC_nominal_specify=off  VC_nominal_value=1  VC_nominal_unit=V
  TripLoad_2 : ee_lib/Passive/RLC Assemblies/Wye-Connected Load  port_option=ee.enum.threePhasePort.composite  parameterization=2  component_structure=1  component_structure_PQ=ee.enum.rlc.structure.R  R=1 Ohm  L=1e-3 H  C=1e-6 F  VRated=230000 V  FRated=50 Hz  P=188000000 W  Qpos=1e2 A*V  Qneg=-1e2 A*V  R_parasitic=0 Ohm  G_parasitic=0 1/Ohm  R_parasitic_PQ=0 Ohm  G_parasitic_PQ=0 1/Ohm  Vmag0=24e3 V  Vang0=0 deg  Freq0=60 Hz  IL_specify=off  IL_priority=High  IL=[0, 0, 0] A  IL_nominal_specify=off  IL_nominal_value=1  IL_nominal_unit=A  VC_specify=off  VC_priority=High  VC=[0, 0, 0] V  VC_nominal_specify=off  VC_nominal_value=1  VC_nominal_unit=V
  VSG_ES1 : Subsystem
  VSG_ES2 : Subsystem
  VSG_ES3 : Subsystem
  VSG_ES4 : Subsystem
  Vabc_ES1 : Subsystem
  Vabc_ES2 : Subsystem
  Vabc_ES3 : Subsystem
  Vabc_ES4 : Subsystem
  Vabc_G1 : Subsystem
  Vabc_G2 : Subsystem
  Vabc_G3 : Subsystem
  Zess_{1..4} (4 alike) : ee_lib/Passive/RLC Assemblies/RLC (Three-Phase)  port_option=ee.enum.threePhasePort.composite  component_structure=4  R=1.587 Ohm  L=0.50516 H  C=1e-6 F  R_parasitic=0 Ohm  G_parasitic=0 1/Ohm  IL_specify=off  IL_priority=High  IL=[0, 0, 0] A  IL_nominal_specify=off  IL_nominal_value=1  IL_nominal_unit=A  VC_specify=off  VC_priority=High  VC=[0, 0, 0] V  VC_nominal_specify=off  VC_nominal_value=1  VC_nominal_unit=V
      settings: InternalSimscapePortConfiguration="{\"Bottom\":[],\"Left\":[{\"id\":\"N1\",\"label\":\"~1\",\"type\":\"foundation.electrical.three_phase\"}],\"Right\":[{\"id\":\"N2\",\"label\":\"~2\",\"type\":\"foundation.electrical.three_phase\"}],\"Top\":[]}"
  Zgen_G1 : ee_lib/Passive/RLC Assemblies/RLC (Three-Phase)  port_option=ee.enum.threePhasePort.composite  component_structure=4  R=1.587 Ohm  L=0.50516 H  C=1e-6 F  R_parasitic=0 Ohm  G_parasitic=0 1/Ohm  IL_specify=off  IL_priority=High  IL=[0, 0, 0] A  IL_nominal_specify=off  IL_nominal_value=1  IL_nominal_unit=A  VC_specify=off  VC_priority=High  VC=[0, 0, 0] V  VC_nominal_specify=off  VC_nominal_value=1  VC_nominal_unit=V
      settings: InternalSimscapePortConfiguration="{\"Bottom\":[],\"Left\":[{\"id\":\"N1\",\"label\":\"~1\",\"type\":\"foundation.electrical.three_phase\"}],\"Right\":[{\"id\":\"N2\",\"label\":\"~2\",\"type\":\"foundation.electrical.three_phase\"}],\"Top\":[]}"
  Zgen_G2 : ee_lib/Passive/RLC Assemblies/RLC (Three-Phase)  port_option=ee.enum.threePhasePort.composite  component_structure=4  R=1.587 Ohm  L=0.50516 H  C=1e-6 F  R_parasitic=0 Ohm  G_parasitic=0 1/Ohm  IL_specify=off  IL_priority=High  IL=[0, 0, 0] A  IL_nominal_specify=off  IL_nominal_value=1  IL_nominal_unit=A  VC_specify=off  VC_priority=High  VC=[0, 0, 0] V  VC_nominal_specify=off  VC_nominal_value=1  VC_nominal_unit=V
      settings: InternalSimscapePortConfiguration="{\"Bottom\":[],\"Left\":[{\"id\":\"N1\",\"label\":\"~1\",\"type\":\"foundation.electrical.three_phase\"}],\"Right\":[{\"id\":\"N2\",\"label\":\"~2\",\"type\":\"foundation.electrical.three_phase\"}],\"Top\":[]}"
  Zgen_G3 : ee_lib/Passive/RLC Assemblies/RLC (Three-Phase)  port_option=ee.enum.threePhasePort.composite  component_structure=4  R=1.587 Ohm  L=0.50516 H  C=1e-6 F  R_parasitic=0 Ohm  G_parasitic=0 1/Ohm  IL_specify=off  IL_priority=High  IL=[0, 0, 0] A  IL_nominal_specify=off  IL_nominal_value=1  IL_nominal_unit=A  VC_specify=off  VC_priority=High  VC=[0, 0, 0] V  VC_nominal_specify=off  VC_nominal_value=1  VC_nominal_unit=V
      settings: InternalSimscapePortConfiguration="{\"Bottom\":[],\"Left\":[{\"id\":\"N1\",\"label\":\"~1\",\"type\":\"foundation.electrical.three_phase\"}],\"Right\":[{\"id\":\"N2\",\"label\":\"~2\",\"type\":\"foundation.electrical.three_phase\"}],\"Top\":[]}"
  Zw_W1 : ee_lib/Passive/RLC Assemblies/RLC (Three-Phase)  port_option=ee.enum.threePhasePort.composite  component_structure=4  R=1.587 Ohm  L=0.50516 H  C=1e-6 F  R_parasitic=0 Ohm  G_parasitic=0 1/Ohm  IL_specify=off  IL_priority=High  IL=[0, 0, 0] A  IL_nominal_specify=off  IL_nominal_value=1  IL_nominal_unit=A  VC_specify=off  VC_priority=High  VC=[0, 0, 0] V  VC_nominal_specify=off  VC_nominal_value=1  VC_nominal_unit=V
      settings: InternalSimscapePortConfiguration="{\"Bottom\":[],\"Left\":[{\"id\":\"N1\",\"label\":\"~1\",\"type\":\"foundation.electrical.three_phase\"}],\"Right\":[{\"id\":\"N2\",\"label\":\"~2\",\"type\":\"foundation.electrical.three_phase\"}],\"Top\":[]}"
  Zw_W2 : ee_lib/Passive/RLC Assemblies/RLC (Three-Phase)  port_option=ee.enum.threePhasePort.composite  component_structure=4  R=1.587 Ohm  L=0.50516 H  C=1e-6 F  R_parasitic=0 Ohm  G_parasitic=0 1/Ohm  IL_specify=off  IL_priority=High  IL=[0, 0, 0] A  IL_nominal_specify=off  IL_nominal_value=1  IL_nominal_unit=A  VC_specify=off  VC_priority=High  VC=[0, 0, 0] V  VC_nominal_specify=off  VC_nominal_value=1  VC_nominal_unit=V
      settings: InternalSimscapePortConfiguration="{\"Bottom\":[],\"Left\":[{\"id\":\"N1\",\"label\":\"~1\",\"type\":\"foundation.electrical.three_phase\"}],\"Right\":[{\"id\":\"N2\",\"label\":\"~2\",\"type\":\"foundation.electrical.three_phase\"}],\"Top\":[]}"
  dD_{1..4} (4 alike) : Constant  Value=0
  dM_{1..4} (4 alike) : Constant  Value=0
  wnt_ES{1..4} (4 alike) : Gain  Gain=314.1593
  wnt_G1 : Gain  Gain=314.1593
  wnt_G2 : Gain  Gain=314.1593
  wnt_G3 : Gain  Gain=314.1593
  wref_{1..4} (4 alike) : Constant  Value=1.0
  wires:
  Clk_G1/1 -> wnt_G1/1
  wnt_G1/1 -> Theta_G1/1
  ConvGen_G1/2(delta) -> Theta_G1/2
  Theta_G1/1 -> Vabc_G1/1(theta)
  Vabc_G1/1(Vabc) -> S2PS_G1/1
  PS2S_G1/1 -> PeGain_G1/1
  PeGain_G1/1 -> ConvGen_G1/1(P_e)
  Clk_G2/1 -> wnt_G2/1
  wnt_G2/1 -> Theta_G2/1
  ConvGen_G2/2(delta) -> Theta_G2/2
  Theta_G2/1 -> Vabc_G2/1(theta)
  Vabc_G2/1(Vabc) -> S2PS_G2/1
  PS2S_G2/1 -> PeGain_G2/1
  PeGain_G2/1 -> ConvGen_G2/1(P_e)
  Clk_G3/1 -> wnt_G3/1
  wnt_G3/1 -> Theta_G3/1
  ConvGen_G3/2(delta) -> Theta_G3/2
  Theta_G3/1 -> Vabc_G3/1(theta)
  Vabc_G3/1(Vabc) -> S2PS_G3/1
  PS2S_G3/1 -> PeGain_G3/1
  PeGain_G3/1 -> ConvGen_G3/1(P_e)
  wref_1/1 -> VSG_ES1/1(omega_ref)
  dM_1/1 -> VSG_ES1/2(delta_M)
  dD_1/1 -> VSG_ES1/3(delta_D)
  Pref_1/1 -> VSG_ES1/4(P_ref)
  Clk_ES1/1 -> wnt_ES1/1
  wnt_ES1/1 -> Theta_ES1/1
  VSG_ES1/2(delta) -> Theta_ES1/2, Log_delta_ES1/1
  Theta_ES1/1 -> Vabc_ES1/1(theta)
  Vabc_ES1/1(Vabc) -> S2PS_ES1/1
  PS2S_ES1/1 -> PeGain_ES1/1
  PeGain_ES1/1 -> VSG_ES1/5(P_e)
  VSG_ES1/1(omega) -> Log_omega_ES1/1
  VSG_ES1/3(P_out) -> Log_P_out_ES1/1
  wref_2/1 -> VSG_ES2/1(omega_ref)
  dM_2/1 -> VSG_ES2/2(delta_M)
  dD_2/1 -> VSG_ES2/3(delta_D)
  Pref_2/1 -> VSG_ES2/4(P_ref)
  Clk_ES2/1 -> wnt_ES2/1
  wnt_ES2/1 -> Theta_ES2/1
  VSG_ES2/2(delta) -> Theta_ES2/2, Log_delta_ES2/1
  Theta_ES2/1 -> Vabc_ES2/1(theta)
  Vabc_ES2/1(Vabc) -> S2PS_ES2/1
  PS2S_ES2/1 -> PeGain_ES2/1
  PeGain_ES2/1 -> VSG_ES2/5(P_e)
  VSG_ES2/1(omega) -> Log_omega_ES2/1
  VSG_ES2/3(P_out) -> Log_P_out_ES2/1
  wref_3/1 -> VSG_ES3/1(omega_ref)
  dM_3/1 -> VSG_ES3/2(delta_M)
  dD_3/1 -> VSG_ES3/3(delta_D)
  Pref_3/1 -> VSG_ES3/4(P_ref)
  Clk_ES3/1 -> wnt_ES3/1
  wnt_ES3/1 -> Theta_ES3/1
  VSG_ES3/2(delta) -> Theta_ES3/2, Log_delta_ES3/1
  Theta_ES3/1 -> Vabc_ES3/1(theta)
  Vabc_ES3/1(Vabc) -> S2PS_ES3/1
  PS2S_ES3/1 -> PeGain_ES3/1
  PeGain_ES3/1 -> VSG_ES3/5(P_e)
  VSG_ES3/1(omega) -> Log_omega_ES3/1
  VSG_ES3/3(P_out) -> Log_P_out_ES3/1
  wref_4/1 -> VSG_ES4/1(omega_ref)
  dM_4/1 -> VSG_ES4/2(delta_M)
  dD_4/1 -> VSG_ES4/3(delta_D)
  Pref_4/1 -> VSG_ES4/4(P_ref)
  Clk_ES4/1 -> wnt_ES4/1
  wnt_ES4/1 -> Theta_ES4/1
  VSG_ES4/2(delta) -> Theta_ES4/2, Log_delta_ES4/1
  Theta_ES4/1 -> Vabc_ES4/1(theta)
  Vabc_ES4/1(Vabc) -> S2PS_ES4/1
  PS2S_ES4/1 -> PeGain_ES4/1
  PeGain_ES4/1 -> VSG_ES4/5(P_e)
  VSG_ES4/1(omega) -> Log_omega_ES4/1
  VSG_ES4/3(P_out) -> Log_P_out_ES4/1
  BrkCtrl_1/1 -> S2PS_Brk1/1
  BrkCtrl_2/1 -> S2PS_Brk2/1
  Clock/1 -> Log_time/1
  connections:
  S2PS_G1/RConn1 -- CVS_G1/LConn1
  CVS_G1/LConn2 -- GND_1/LConn1
  CVS_G1/RConn1 -- Zgen_G1/LConn1
  Zgen_G1/RConn1 -- PSens_G1/LConn1
  PSens_G1/LConn2 -- PS2S_G1/LConn1
  S2PS_G2/RConn1 -- CVS_G2/LConn1
  CVS_G2/LConn2 -- GND_2/LConn1
  CVS_G2/RConn1 -- Zgen_G2/LConn1
  Zgen_G2/RConn1 -- PSens_G2/LConn1
  PSens_G2/LConn2 -- PS2S_G2/LConn1
  S2PS_G3/RConn1 -- CVS_G3/LConn1
  CVS_G3/LConn2 -- GND_3/LConn1
  CVS_G3/RConn1 -- Zgen_G3/LConn1
  Zgen_G3/RConn1 -- PSens_G3/LConn1
  PSens_G3/LConn2 -- PS2S_G3/LConn1
  PVS_W1/LConn1 -- GND_4/LConn1
  PVS_W1/RConn1 -- Zw_W1/LConn1
  PVS_W2/LConn1 -- GND_5/LConn1
  PVS_W2/RConn1 -- Zw_W2/LConn1
  S2PS_ES1/RConn1 -- CVS_ES1/LConn1
  CVS_ES1/LConn2 -- GND_6/LConn1
  CVS_ES1/RConn1 -- Zess_1/LConn1
  Zess_1/RConn1 -- PSens_ES1/LConn1
  PSens_ES1/LConn2 -- PS2S_ES1/LConn1
  S2PS_ES2/RConn1 -- CVS_ES2/LConn1
  CVS_ES2/LConn2 -- GND_7/LConn1
  CVS_ES2/RConn1 -- Zess_2/LConn1
  Zess_2/RConn1 -- PSens_ES2/LConn1
  PSens_ES2/LConn2 -- PS2S_ES2/LConn1
  S2PS_ES3/RConn1 -- CVS_ES3/LConn1
  CVS_ES3/LConn2 -- GND_8/LConn1
  CVS_ES3/RConn1 -- Zess_3/LConn1
  Zess_3/RConn1 -- PSens_ES3/LConn1
  PSens_ES3/LConn2 -- PS2S_ES3/LConn1
  S2PS_ES4/RConn1 -- CVS_ES4/LConn1
  CVS_ES4/LConn2 -- GND_9/LConn1
  CVS_ES4/RConn1 -- Zess_4/LConn1
  Zess_4/RConn1 -- PSens_ES4/LConn1
  PSens_ES4/LConn2 -- PS2S_ES4/LConn1
  L_1_5/LConn1 -- PSens_G1/RConn1 -- SolverConfig/RConn1
  L_1_5/LConn2 -- GND_10/LConn1
  L_1_5/RConn2 -- GND_11/LConn1
  PSens_G2/RConn1 -- L_2_6/LConn1
  L_2_6/LConn2 -- GND_12/LConn1
  L_2_6/RConn2 -- GND_13/LConn1
  PSens_G3/RConn1 -- L_3_10/LConn1
  L_3_10/LConn2 -- GND_14/LConn1
  L_3_10/RConn2 -- GND_15/LConn1
  Zw_W1/RConn1 -- L_4_9/LConn1
  L_4_9/LConn2 -- GND_16/LConn1
  L_4_9/RConn2 -- GND_17/LConn1
  L_5_6a/LConn1 -- L_1_5/RConn1 -- L_5_6b/LConn1
  L_5_6a/RConn1 -- L_2_6/RConn1 -- L_5_6b/RConn1 -- L_6_7a/LConn1 -- L_6_7b/LConn1
  L_5_6a/LConn2 -- GND_18/LConn1
  L_5_6a/RConn2 -- GND_19/LConn1
  L_5_6b/LConn2 -- GND_20/LConn1
  L_5_6b/RConn2 -- GND_21/LConn1
  L_6_7a/LConn2 -- GND_22/LConn1
  L_6_7a/RConn2 -- GND_23/LConn1
  L_6_7b/RConn1 -- L_6_7a/RConn1 -- L_7_8a/LConn1 -- L_7_8b/LConn1 -- L_7_8c/LConn1 -- L_7_12/LConn1 -- Load7/LConn1 -- Shunt7/LConn1
  L_6_7b/LConn2 -- GND_24/LConn1
  L_6_7b/RConn2 -- GND_25/LConn1
  L_7_8a/LConn2 -- GND_26/LConn1
  L_7_8a/RConn2 -- GND_27/LConn1
  L_7_8b/RConn1 -- L_7_8a/RConn1 -- L_7_8c/RConn1 -- L_8_9a/LConn1 -- L_8_9b/LConn1 -- L_8_16/LConn1 -- L_8_W2/LConn1
  L_7_8b/LConn2 -- GND_28/LConn1
  L_7_8b/RConn2 -- GND_29/LConn1
  L_7_8c/LConn2 -- GND_30/LConn1
  L_7_8c/RConn2 -- GND_31/LConn1
  L_8_9a/RConn1 -- L_4_9/RConn1 -- L_8_9b/RConn1 -- L_9_10a/LConn1 -- L_9_10b/LConn1 -- L_9_15/LConn1 -- Load9/LConn1 -- Shunt9/LConn1
  L_8_9a/LConn2 -- GND_32/LConn1
  L_8_9a/RConn2 -- GND_33/LConn1
  L_8_9b/LConn2 -- GND_34/LConn1
  L_8_9b/RConn2 -- GND_35/LConn1
  L_9_10a/RConn1 -- L_3_10/RConn1 -- L_9_10b/RConn1 -- L_10_14/LConn1
  L_9_10a/LConn2 -- GND_36/LConn1
  L_9_10a/RConn2 -- GND_37/LConn1
  L_9_10b/LConn2 -- GND_38/LConn1
  L_9_10b/RConn2 -- GND_39/LConn1
  PSens_ES1/RConn1 -- L_7_12/RConn1
  L_7_12/LConn2 -- GND_40/LConn1
  L_7_12/RConn2 -- GND_41/LConn1
  PSens_ES2/RConn1 -- L_8_16/RConn1
  L_8_16/LConn2 -- GND_42/LConn1
  L_8_16/RConn2 -- GND_43/LConn1
  L_10_14/RConn1 -- PSens_ES3/RConn1 -- Breaker_1/LConn2
  L_10_14/LConn2 -- GND_44/LConn1
  L_10_14/RConn2 -- GND_45/LConn1
  L_9_15/RConn1 -- PSens_ES4/RConn1 -- Breaker_2/LConn2
  L_9_15/LConn2 -- GND_46/LConn1
  L_9_15/RConn2 -- GND_47/LConn1
  Zw_W2/RConn1 -- L_8_W2/RConn1
  L_8_W2/LConn2 -- GND_48/LConn1
  L_8_W2/RConn2 -- GND_49/LConn1
  Load7/RConn1 -- GND_50/LConn1
  Load9/RConn1 -- GND_51/LConn1
  Shunt7/RConn1 -- GND_52/LConn1
  Shunt9/RConn1 -- GND_53/LConn1
  S2PS_Brk1/RConn1 -- Breaker_1/LConn1
  Breaker_1/RConn1 -- TripLoad_1/LConn1
  TripLoad_1/RConn1 -- GND_54/LConn1
  S2PS_Brk2/RConn1 -- Breaker_2/LConn1
  Breaker_2/RConn1 -- TripLoad_2/LConn1
  TripLoad_2/RConn1 -- GND_55/LConn1

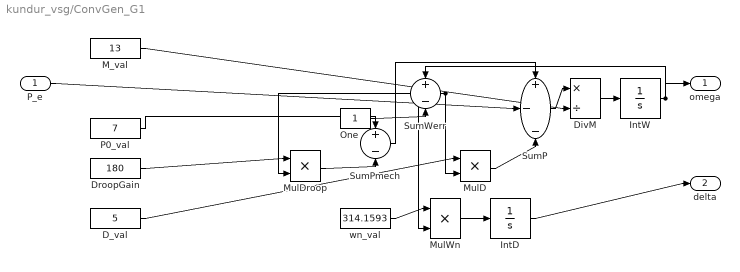
== system kundur_vsg/ConvGen_G1 ==
  P_e : Inport
  D_val : Constant  Value=5
  DivM : Product  Inputs=*/
  DroopGain : Constant  Value=180
  IntD : Integrator
  IntW : Integrator  InitialCondition=1.0  LimitOutput=on  UpperSaturationLimit=1.1  LowerSaturationLimit=0.9
  M_val : Constant  Value=13
  MulD : Product  Inputs=**
  MulDroop : Product  Inputs=**
  MulWn : Product  Inputs=**
  One : Constant
  P0_val : Constant  Value=7
  SumP : Sum  Inputs=+--
  SumPmech : Sum  Inputs=+-
  SumWerr : Sum  Inputs=+-
  wn_val : Constant  Value=314.1593
  omega : Outport
  delta : Outport  Port=2
  wires:
  IntW/1 -> omega/1, SumWerr/1
  One/1 -> SumWerr/2
  DroopGain/1 -> MulDroop/1
  SumWerr/1 -> MulDroop/2, MulD/2, MulWn/2
  P0_val/1 -> SumPmech/1
  MulDroop/1 -> SumPmech/2
  D_val/1 -> MulD/1
  SumPmech/1 -> SumP/1
  P_e/1 -> SumP/2
  MulD/1 -> SumP/3
  SumP/1 -> DivM/1
  M_val/1 -> DivM/2
  DivM/1 -> IntW/1
  wn_val/1 -> MulWn/1
  MulWn/1 -> IntD/1
  IntD/1 -> delta/1

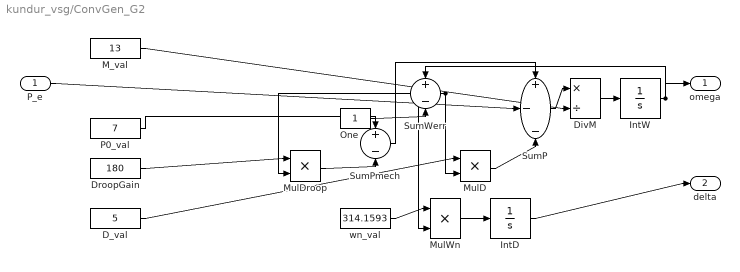
== system kundur_vsg/ConvGen_G2 ==
  P_e : Inport
  D_val : Constant  Value=5
  DivM : Product  Inputs=*/
  DroopGain : Constant  Value=180
  IntD : Integrator  InitialCondition=-0.043633
  IntW : Integrator  InitialCondition=1.0  LimitOutput=on  UpperSaturationLimit=1.1  LowerSaturationLimit=0.9
  M_val : Constant  Value=13
  MulD : Product  Inputs=**
  MulDroop : Product  Inputs=**
  MulWn : Product  Inputs=**
  One : Constant
  P0_val : Constant  Value=7
  SumP : Sum  Inputs=+--
  SumPmech : Sum  Inputs=+-
  SumWerr : Sum  Inputs=+-
  wn_val : Constant  Value=314.1593
  omega : Outport
  delta : Outport  Port=2
  wires:
  IntW/1 -> omega/1, SumWerr/1
  One/1 -> SumWerr/2
  DroopGain/1 -> MulDroop/1
  SumWerr/1 -> MulDroop/2, MulD/2, MulWn/2
  P0_val/1 -> SumPmech/1
  MulDroop/1 -> SumPmech/2
  D_val/1 -> MulD/1
  SumPmech/1 -> SumP/1
  P_e/1 -> SumP/2
  MulD/1 -> SumP/3
  SumP/1 -> DivM/1
  M_val/1 -> DivM/2
  DivM/1 -> IntW/1
  wn_val/1 -> MulWn/1
  MulWn/1 -> IntD/1
  IntD/1 -> delta/1

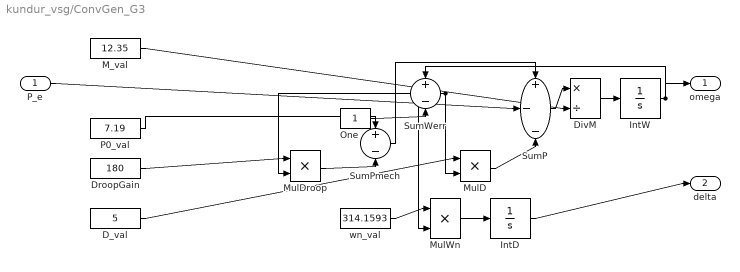
== system kundur_vsg/ConvGen_G3 ==
  P_e : Inport
  D_val : Constant  Value=5
  DivM : Product  Inputs=*/
  DroopGain : Constant  Value=180
  IntD : Integrator  InitialCondition=-0.087266
  IntW : Integrator  InitialCondition=1.0  LimitOutput=on  UpperSaturationLimit=1.1  LowerSaturationLimit=0.9
  M_val : Constant  Value=12.35
  MulD : Product  Inputs=**
  MulDroop : Product  Inputs=**
  MulWn : Product  Inputs=**
  One : Constant
  P0_val : Constant  Value=7.19
  SumP : Sum  Inputs=+--
  SumPmech : Sum  Inputs=+-
  SumWerr : Sum  Inputs=+-
  wn_val : Constant  Value=314.1593
  omega : Outport
  delta : Outport  Port=2
  wires:
  IntW/1 -> omega/1, SumWerr/1
  One/1 -> SumWerr/2
  DroopGain/1 -> MulDroop/1
  SumWerr/1 -> MulDroop/2, MulD/2, MulWn/2
  P0_val/1 -> SumPmech/1
  MulDroop/1 -> SumPmech/2
  D_val/1 -> MulD/1
  SumPmech/1 -> SumP/1
  P_e/1 -> SumP/2
  MulD/1 -> SumP/3
  SumP/1 -> DivM/1
  M_val/1 -> DivM/2
  DivM/1 -> IntW/1
  wn_val/1 -> MulWn/1
  MulWn/1 -> IntD/1
  IntD/1 -> delta/1

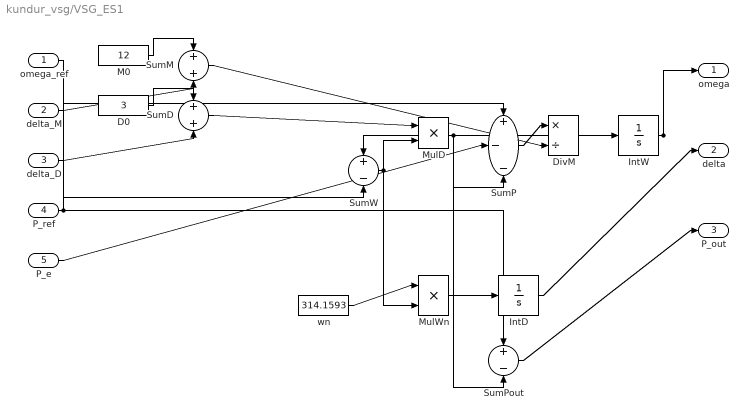
== system kundur_vsg/VSG_ES1 ==
  omega_ref : Inport
  delta_M : Inport  Port=2
  delta_D : Inport  Port=3
  P_ref : Inport  Port=4
  P_e : Inport  Port=5
  D0 : Constant  Value=3
  DivM : Product  Inputs=*/
  IntD : Integrator  InitialCondition=-0.05236
  IntW : Integrator  InitialCondition=1.0  LimitOutput=on  UpperSaturationLimit=1.1  LowerSaturationLimit=0.9
  M0 : Constant  Value=12
  MulD : Product  Inputs=**
  MulWn : Product  Inputs=**
  SumD : Sum
  SumM : Sum
  SumP : Sum  Inputs=+--
  SumPout : Sum  Inputs=+-
  SumW : Sum  Inputs=+-
  wn : Constant  Value=314.1593
  omega : Outport
  delta : Outport  Port=2
  P_out : Outport  Port=3
  wires:
  M0/1 -> SumM/1
  delta_M/1 -> SumM/2
  D0/1 -> SumD/1
  delta_D/1 -> SumD/2
  IntW/1 -> omega/1, SumW/1
  omega_ref/1 -> SumW/2
  SumD/1 -> MulD/1
  SumW/1 -> MulD/2, MulWn/2
  P_ref/1 -> SumP/1, SumPout/1
  P_e/1 -> SumP/2
  MulD/1 -> SumP/3, SumPout/2
  SumP/1 -> DivM/1
  SumM/1 -> DivM/2
  DivM/1 -> IntW/1
  wn/1 -> MulWn/1
  MulWn/1 -> IntD/1
  IntD/1 -> delta/1
  SumPout/1 -> P_out/1

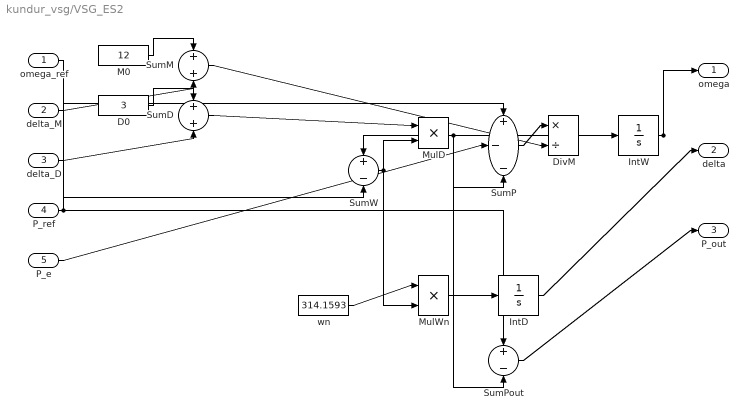
== system kundur_vsg/VSG_ES2 ==
  omega_ref : Inport
  delta_M : Inport  Port=2
  delta_D : Inport  Port=3
  P_ref : Inport  Port=4
  P_e : Inport  Port=5
  D0 : Constant  Value=3
  DivM : Product  Inputs=*/
  IntD : Integrator  InitialCondition=-0.07854
  IntW : Integrator  InitialCondition=1.0  LimitOutput=on  UpperSaturationLimit=1.1  LowerSaturationLimit=0.9
  M0 : Constant  Value=12
  MulD : Product  Inputs=**
  MulWn : Product  Inputs=**
  SumD : Sum
  SumM : Sum
  SumP : Sum  Inputs=+--
  SumPout : Sum  Inputs=+-
  SumW : Sum  Inputs=+-
  wn : Constant  Value=314.1593
  omega : Outport
  delta : Outport  Port=2
  P_out : Outport  Port=3
  wires:
  M0/1 -> SumM/1
  delta_M/1 -> SumM/2
  D0/1 -> SumD/1
  delta_D/1 -> SumD/2
  IntW/1 -> omega/1, SumW/1
  omega_ref/1 -> SumW/2
  SumD/1 -> MulD/1
  SumW/1 -> MulD/2, MulWn/2
  P_ref/1 -> SumP/1, SumPout/1
  P_e/1 -> SumP/2
  MulD/1 -> SumP/3, SumPout/2
  SumP/1 -> DivM/1
  SumM/1 -> DivM/2
  DivM/1 -> IntW/1
  wn/1 -> MulWn/1
  MulWn/1 -> IntD/1
  IntD/1 -> delta/1
  SumPout/1 -> P_out/1
